simulink model "DCM_Due"  (R2020a)
settings: Solver=FixedStepAuto  StartTime=0.0  StopTime=10  RelTol=1e-3  EnableMultiTasking=on
undefined symbols (not defined in the file): Iumax, J, Ki_I, Kp_I, Kp_W, Kphi, Lu, Ru, T, Ubat
libraries: arduinolib x12, simulink x8, powerlib_meascontrol x1
settings Model: SimulationMode=external  SILPILModeSetting=veronly  ExtModeTrigDuration=2  Creator=Nguyen Tung  LastModifiedBy=Nguyen Tung
settings OptimizationCC: StrengthReduction=on  PassReuseOutputArgsAs=Individual arguments  ZeroExternalMemoryAtStartup=off  ZeroInternalMemoryAtStartup=off  MaxStackSize=64  OptimizeBlockOrder=speed  OptimizationPriority=Speed  OptimizationCustomize=off  MultiThreadedLoops=on  EfficientTunableParamExpr=on
settings DebuggingCC: ParameterTunabilityLossMsg=error
settings HardwareCC: ProdBitPerPointer=32  ProdBitPerSizeT=32  ProdBitPerPtrDiffT=32  ProdLargestAtomicInteger=Long  ProdLargestAtomicFloat=Double  ProdWordSize=32  ProdHWDeviceType=ARM Compatible->ARM Cortex
settings SFSimCC: MATLABDynamicMemAlloc=off
settings RTWCC: SystemTargetFile=ert.tlc  HardwareBoard=Arduino Due  TLCOptions=-aInlineSetEventsForThisBaseRateFcn=TLC_FALSE -aSuppressMultiTaskScheduler=TLC_FALSE -aRateBasedStepFcn=1  TemplateMakefile=ert_default_tmf  GenerateReport=on  Toolchain=Arduino ARM  BuildConfiguration=Faster Runs
settings CodeAppCC: ForceParamTrailComments=on  IgnoreCustomStorageClasses=off  OperatorAnnotations=on  SimulinkDataObjDesc=on  SFDataObjDesc=on  InsertBlockDesc=on
settings ERTTargetCC: SupportContinuousTime=on  SupportVariableSizeSignals=on  ExtMode=on  ExtModeTransport=3  ExtModeStaticAlloc=on  ExtModeStaticAllocSize=24576  ExtModeMexFile=ext_xcp  ExtModeMexArgs=0 5 115200  ExtModeIntrfLevel=Level2 - Open

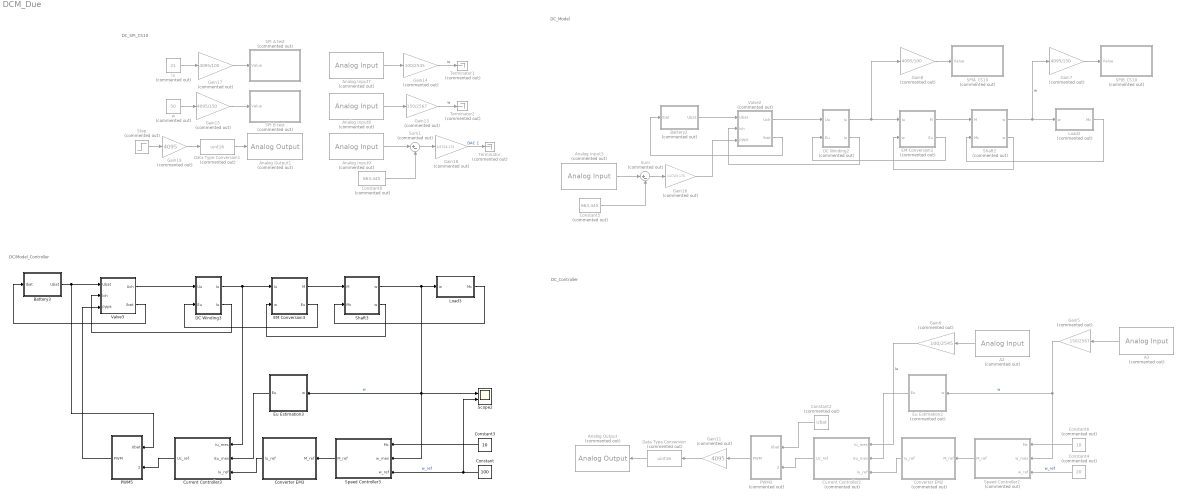
== system DCM_Due ==
  note: DC_Controller
  note: DC/Model_Controller
  note: DC_SPI_CS10
  note: DC_Model
  A2 : arduinolib/Analog Input  Commented=on  pinNumber=2  ReadResultsOnly=off  ConversionTriggerSource=Software  ExternalTriggerType=uint32( 0 )  OutputDataType=uint16  EnableConversionCompleteNotify=off  EnableOuputStatus=off  SampleTime=T  blockPlatform=arduino
  A3 : arduinolib/Analog Input  Commented=on  pinNumber=3  ReadResultsOnly=off  ConversionTriggerSource=Software  ExternalTriggerType=uint32( 0 )  OutputDataType=uint16  EnableConversionCompleteNotify=off  EnableOuputStatus=off  SampleTime=T  blockPlatform=arduino
  Analog Input3 : arduinolib/Analog Input  Commented=on  pinNumber=1  ReadResultsOnly=off  ConversionTriggerSource=Software  ExternalTriggerType=uint32( 0 )  OutputDataType=uint16  EnableConversionCompleteNotify=off  EnableOuputStatus=off  SampleTime=T  blockPlatform=arduino
  Analog Input7 : arduinolib/Analog Input  Commented=on  pinNumber=2  ReadResultsOnly=off  ConversionTriggerSource=Software  ExternalTriggerType=uint32( 0 )  OutputDataType=uint16  EnableConversionCompleteNotify=off  EnableOuputStatus=off  SampleTime=T  blockPlatform=arduino
  Analog Input8 : arduinolib/Analog Input  Commented=on  pinNumber=3  ReadResultsOnly=off  ConversionTriggerSource=Software  ExternalTriggerType=uint32( 0 )  OutputDataType=uint16  EnableConversionCompleteNotify=off  EnableOuputStatus=off  SampleTime=T  blockPlatform=arduino
  Analog Input9 : arduinolib/Analog Input  Commented=on  pinNumber=1  ReadResultsOnly=off  ConversionTriggerSource=Software  ExternalTriggerType=uint32( 0 )  OutputDataType=uint16  EnableConversionCompleteNotify=off  EnableOuputStatus=off  SampleTime=T  blockPlatform=arduino
  Analog Output : arduinolib/Analog Output  Commented=on  DACpin=DAC1  blockPlatform=arduino
      settings: SourceProductBaseCode=ARDUINO
  Analog Output1 : arduinolib/Analog Output  Commented=on  DACpin=DAC1  blockPlatform=arduino
      settings: SourceProductBaseCode=ARDUINO
  Battery2 : Subsystem  Commented=on  AncestorBlock=simulink/REM/SE
      mask Display:
      | plot(0,0,100,100, 1.2*[50,57.68,60.77,63.08,64.97,66.58,68,69.26,70.4, 	71.42,72.36,78.28,80,78.28,72.36,71.42,70.4, 	69.26,68,66.58,64.97,63.08,60.77,57.68,50,42.32, 	39.23,36.92,35.03,33.42,32,30.74,29.6,28.58, 	27.64,21.72,20,21.72,27.64,28.58,29.6,30.74,32, 	33.42,35.03,36.92,39.23,42.32,50]-10, 1.2*[20,21,22,23,24,25,26,27,28,29,30,40,50,60,70,71,72, 	73,74,75,76,77,78,79,80,79,78,77,76,75,74,73,72, 	71,70,60,50,40,30,29,28,27,26,25,24,23,22,21,20]-10)
      | disp('ES')
  Battery3 : Subsystem  AncestorBlock=simulink/REM/SE
      mask Display:
      | plot(0,0,100,100, 1.2*[50,57.68,60.77,63.08,64.97,66.58,68,69.26,70.4, 	71.42,72.36,78.28,80,78.28,72.36,71.42,70.4, 	69.26,68,66.58,64.97,63.08,60.77,57.68,50,42.32, 	39.23,36.92,35.03,33.42,32,30.74,29.6,28.58, 	27.64,21.72,20,21.72,27.64,28.58,29.6,30.74,32, 	33.42,35.03,36.92,39.23,42.32,50]-10, 1.2*[20,21,22,23,24,25,26,27,28,29,30,40,50,60,70,71,72, 	73,74,75,76,77,78,79,80,79,78,77,76,75,74,73,72, 	71,70,60,50,40,30,29,28,27,26,25,24,23,22,21,20]-10)
      | disp('ES')
  Constant : Constant  Value=100  SampleTime=T
  Constant2 : Constant  Commented=on  Value=Ubat
  Constant3 : Constant  Value=10  SampleTime=T
  Constant4 : Constant  Commented=on  Value=20
  Constant5 : Constant  Commented=on  Value=663.445
  Constant6 : Constant  Commented=on  Value=10
  Constant8 : Constant  Commented=on  Value=663.445
  Converter EM2 : Subsystem  Commented=on  AncestorBlock=simulink/SMC/Inversion EC avec mesure
      mask Display: plot(0,0,100,100,[10,30,90,70,10],[90,10,10,90,90])
  Converter EM3 : Subsystem  AncestorBlock=simulink/SMC/Inversion EC avec mesure
      mask Display: plot(0,0,100,100,[10,30,90,70,10],[90,10,10,90,90])
  Current Controller2 : Subsystem  Commented=on  AncestorBlock=simulink/SMC/Asservissement Correcteur IP
      mask Display: plot(0,0,100,100, [10,30,90,70,10,90],[90,10,10,90,90,10])
  Current Controller3 : Subsystem  AncestorBlock=simulink/SMC/Asservissement Correcteur IP
      mask Display: plot(0,0,100,100, [10,30,90,70,10,90],[90,10,10,90,90,10])
  DC Winding2 : Subsystem  Commented=on  AncestorBlock=simulink/REM/EA  mask(CM){}
      mask Display: plot(0,0,100,100,[10,10,90,90,10],[90,10,10,90,90], [10,90],[10,90])
  DC Winding3 : Subsystem  AncestorBlock=simulink/REM/EA  mask(CM){}
      mask Display: plot(0,0,100,100,[10,10,90,90,10],[90,10,10,90,90], [10,90],[10,90])
  Data Type Conversion : DataTypeConversion  Commented=on  OutDataTypeStr=uint16  RndMeth=Nearest
  Data Type Conversion1 : DataTypeConversion  Commented=on  OutDataTypeStr=uint16
  EM Conversion2 : Subsystem  Commented=on  AncestorBlock=simulink/REM/EC EM
      mask Display: plot(0,0,100,100, 1.4*[50,57.68,60.77,63.08,64.97,66.58,68,69.26,70.4, 	71.42,72.36,78.28,80,78.28,72.36,71.42,70.4, 	69.26,68,66.58,64.97,63.08,60.77,57.68,50,42.32, 	39.23,36.92,35.03,33.42,32,30.74,29.6,28.58, 	27.64,21.72,20,21.72,27.64,28.58,29.6,30.74,32, 	33.42,35.03,36.92,39.23,42.32,50]-20, 1.4*[20,21,22,23,24,25,26,27,28,29,30,40,50,60,70,71,72, 	73,74,75,76,77,78,79,80,79,78,77,76,75,74,73,72, 	71,70,60,50,40,30,29,28,27,26,25,24,23,22,21,20]-20)
  EM Conversion3 : Subsystem  AncestorBlock=simulink/REM/EC EM
      mask Display: plot(0,0,100,100, 1.4*[50,57.68,60.77,63.08,64.97,66.58,68,69.26,70.4, 	71.42,72.36,78.28,80,78.28,72.36,71.42,70.4, 	69.26,68,66.58,64.97,63.08,60.77,57.68,50,42.32, 	39.23,36.92,35.03,33.42,32,30.74,29.6,28.58, 	27.64,21.72,20,21.72,27.64,28.58,29.6,30.74,32, 	33.42,35.03,36.92,39.23,42.32,50]-20, 1.4*[20,21,22,23,24,25,26,27,28,29,30,40,50,60,70,71,72, 	73,74,75,76,77,78,79,80,79,78,77,76,75,74,73,72, 	71,70,60,50,40,30,29,28,27,26,25,24,23,22,21,20]-20)
  Eu Estimation2 : Subsystem  Commented=on  AncestorBlock=simulink/REM/EC EM
      mask Display: plot(0,0,100,100, 1.4*[50,57.68,60.77,63.08,64.97,66.58,68,69.26,70.4, 	71.42,72.36,78.28,80,78.28,72.36,71.42,70.4, 	69.26,68,66.58,64.97,63.08,60.77,57.68,50,42.32, 	39.23,36.92,35.03,33.42,32,30.74,29.6,28.58, 	27.64,21.72,20,21.72,27.64,28.58,29.6,30.74,32, 	33.42,35.03,36.92,39.23,42.32,50]-20, 1.4*[20,21,22,23,24,25,26,27,28,29,30,40,50,60,70,71,72, 	73,74,75,76,77,78,79,80,79,78,77,76,75,74,73,72, 	71,70,60,50,40,30,29,28,27,26,25,24,23,22,21,20]-20)
  Eu Estimation3 : Subsystem  AncestorBlock=simulink/REM/EC EM
      mask Display: plot(0,0,100,100, 1.4*[50,57.68,60.77,63.08,64.97,66.58,68,69.26,70.4, 	71.42,72.36,78.28,80,78.28,72.36,71.42,70.4, 	69.26,68,66.58,64.97,63.08,60.77,57.68,50,42.32, 	39.23,36.92,35.03,33.42,32,30.74,29.6,28.58, 	27.64,21.72,20,21.72,27.64,28.58,29.6,30.74,32, 	33.42,35.03,36.92,39.23,42.32,50]-20, 1.4*[20,21,22,23,24,25,26,27,28,29,30,40,50,60,70,71,72, 	73,74,75,76,77,78,79,80,79,78,77,76,75,74,73,72, 	71,70,60,50,40,30,29,28,27,26,25,24,23,22,21,20]-20)
  Gain11 : Gain  Commented=on  Gain=4095
  Gain13 : Gain  Commented=on  Gain=150/2567
  Gain14 : Gain  Commented=on  Gain=100/2545
  Gain15 : Gain  Commented=on  Gain=4095/150
  Gain16 : Gain  Commented=on  Gain=1/2723.175
  Gain17 : Gain  Commented=on  Gain=4095/100
  Gain18 : Gain  Commented=on  Gain=1/2723.175
  Gain19 : Gain  Commented=on  Gain=4095
  Gain5 : Gain  Commented=on  Gain=150/2567
  Gain6 : Gain  Commented=on  Gain=100/2545
  Gain7 : Gain  Commented=on  Gain=4095/150
  Gain8 : Gain  Commented=on  Gain=4095/100
  Iu : Constant  Commented=on  Value=21  SampleTime=T
  Load2 : Subsystem  Commented=on  AncestorBlock=simulink/REM/SE
      mask Display:
      | plot(0,0,100,100, 1.2*[50,57.68,60.77,63.08,64.97,66.58,68,69.26,70.4, 	71.42,72.36,78.28,80,78.28,72.36,71.42,70.4, 	69.26,68,66.58,64.97,63.08,60.77,57.68,50,42.32, 	39.23,36.92,35.03,33.42,32,30.74,29.6,28.58, 	27.64,21.72,20,21.72,27.64,28.58,29.6,30.74,32, 	33.42,35.03,36.92,39.23,42.32,50]-10, 1.2*[20,21,22,23,24,25,26,27,28,29,30,40,50,60,70,71,72, 	73,74,75,76,77,78,79,80,79,78,77,76,75,74,73,72, 	71,70,60,50,40,30,29,28,27,26,25,24,23,22,21,20]-10)
      | disp('MS')
  Load3 : Subsystem  AncestorBlock=simulink/REM/SE
      mask Display:
      | plot(0,0,100,100, 1.2*[50,57.68,60.77,63.08,64.97,66.58,68,69.26,70.4, 	71.42,72.36,78.28,80,78.28,72.36,71.42,70.4, 	69.26,68,66.58,64.97,63.08,60.77,57.68,50,42.32, 	39.23,36.92,35.03,33.42,32,30.74,29.6,28.58, 	27.64,21.72,20,21.72,27.64,28.58,29.6,30.74,32, 	33.42,35.03,36.92,39.23,42.32,50]-10, 1.2*[20,21,22,23,24,25,26,27,28,29,30,40,50,60,70,71,72, 	73,74,75,76,77,78,79,80,79,78,77,76,75,74,73,72, 	71,70,60,50,40,30,29,28,27,26,25,24,23,22,21,20]-10)
      | disp('MS')
  PWM3 : Subsystem  Commented=on  AncestorBlock=simulink/SMC/Inversion EC avec mesure
      mask Display: plot(0,0,100,100,[10,30,90,70,10],[90,10,10,90,90])
  PWM5 : Subsystem  AncestorBlock=simulink/SMC/Inversion EC avec mesure
      mask Display: plot(0,0,100,100,[10,30,90,70,10],[90,10,10,90,90])
  SPI A test : Subsystem  Commented=on
  SPI B test : Subsystem  Commented=on
  SPIA_CS10 : Subsystem  Commented=on
  SPIB_CS10 : Subsystem  Commented=on
  Scope2 : Scope  NumInputPorts=2
  Shaft2 : Subsystem  Commented=on  AncestorBlock=simulink/REM/EA  mask(CM){}
      mask Display: plot(0,0,100,100,[10,10,90,90,10],[90,10,10,90,90], [10,90],[10,90])
  Shaft3 : Subsystem  AncestorBlock=simulink/REM/EA  mask(CM){}
      mask Display: plot(0,0,100,100,[10,10,90,90,10],[90,10,10,90,90], [10,90],[10,90])
  Speed Controller2 : Subsystem  Commented=on  AncestorBlock=simulink/SMC/Asservissement Correcteur IP
      mask Display: plot(0,0,100,100, [10,30,90,70,10,90],[90,10,10,90,90,10])
  Speed Controller3 : Subsystem  AncestorBlock=simulink/SMC/Asservissement Correcteur IP
      mask Display: plot(0,0,100,100, [10,30,90,70,10,90],[90,10,10,90,90,10])
  Step : Step  Commented=on  Time=5  SampleTime=0
  Sum : Sum  Commented=on  Inputs=|+-
  Sum1 : Sum  Commented=on  Inputs=|+-
  Terminator : Terminator  Commented=on
  Terminator1 : Terminator  Commented=on
  Terminator2 : Terminator  Commented=on
  Valve2 : Subsystem  Commented=on  AncestorBlock=simulink/REM/EC Elec  mask(Hacheur){}
      mask Display: plot(0,0,100,100,[10,10,90,90,10],[90,10,10,90,90])
  Valve3 : Subsystem  AncestorBlock=simulink/REM/EC Elec  mask(Hacheur){}
      mask Display: plot(0,0,100,100,[10,10,90,90,10],[90,10,10,90,90])
  w : Constant  Commented=on  Value=50  SampleTime=T
  wires:
  Valve2/1(Uch) -> DC Winding2/1(Uu)
  Speed Controller2/1(M_ref) -> Converter EM2/1(M_ref)
  Valve3/2(Ibat) -> Battery3/1(Ibat)
  A2/1 -> Gain6/1
  Iu/1 -> Gain17/1
  Gain5/1 -> Eu Estimation2/1(w), Speed Controller2/2(w_mes)  "w"
  PWM3/1(PWM) -> Gain11/1
  EM Conversion3/1(M) -> Shaft3/1(M)
  DC Winding2/2("Iu ") -> Valve2/2(Ich)
  Converter EM3/1(Iu_ref) -> Current Controller3/3(Iu_ref)
  Converter EM2/1(Iu_ref) -> Current Controller2/3(Iu_ref)
  Battery3/1(Ubat) -> Valve3/1(Ubat), PWM5/1(Ubat)
  Eu Estimation2/1(Eu) -> Current Controller2/2(Eu_mes)
  Gain16/1 -> Valve2/3(PWM)
  Shaft2/2("w ") -> EM Conversion2/2(w)
  EM Conversion2/2(Eu) -> DC Winding2/2(Eu)
  Analog Input3/1 -> Sum/1
  Gain18/1 -> Terminator/1  "DAC 1"
  Shaft3/1(w) -> Speed Controller3/2(w_mes), Scope2/1, Eu Estimation3/1(w), Load3/1(w)  "w"
  Constant3/1 -> Speed Controller3/1(Mc)
  Gain11/1 -> Data Type Conversion/1
  Speed Controller3/1(M_ref) -> Converter EM3/1(M_ref)
  Current Controller3/1(Uc_ref) -> PWM5/2(Uch_ref)
  DC Winding3/1(Iu) -> EM Conversion3/1(Iu), Current Controller3/1(Iu_mes)
  Data Type Conversion/1 -> Analog Output/1
  Shaft2/1(w) -> Gain7/1, Load2/1(w)  "w"
  PWM5/1(PWM) -> Valve3/3(PWM)
  Constant/1 -> Speed Controller3/3(w_ref), Scope2/2  "w_ref"
  Constant6/1 -> Speed Controller2/1(Mc)
  Step/1 -> Gain19/1
  Data Type Conversion1/1 -> Analog Output1/1
  EM Conversion3/2(Eu) -> DC Winding3/2(Eu)
  Constant8/1 -> Sum1/2
  Gain19/1 -> Data Type Conversion1/1
  A3/1 -> Gain5/1
  Valve2/2(Ibat) -> Battery2/1(Ibat)
  Valve3/1(Uch) -> DC Winding3/1(Uu)
  Constant5/1 -> Sum/2
  DC Winding2/1(Iu) -> Gain8/1, EM Conversion2/1(Iu)
  Constant4/1 -> Speed Controller2/3(w_ref)  "w_ref"
  EM Conversion2/1(M) -> Shaft2/1(M)
  Gain8/1 -> SPIA_CS10/1(Value)
  Load3/1(Mc) -> Shaft3/2(Mc)
  DC Winding3/2("Iu ") -> Valve3/2(Ich)
  Shaft3/2("w ") -> EM Conversion3/2(w)
  Load2/1(Mc) -> Shaft2/2(Mc)
  Gain14/1 -> Terminator1/1  "iu"
  Sum1/1 -> Gain18/1
  Analog Input7/1 -> Gain14/1
  Sum/1 -> Gain16/1
  Gain7/1 -> SPIB_CS10/1(Value)
  Constant2/1 -> PWM3/1(Ubat)
  Analog Input9/1 -> Sum1/1
  Gain17/1 -> SPI A test/1(Value)
  Current Controller2/1(Uc_ref) -> PWM3/2(Uch_ref)
  Battery2/1(Ubat) -> Valve2/1(Ubat)
  Gain6/1 -> Current Controller2/1(Iu_mes)  "Iu"
  Eu Estimation3/1(Eu) -> Current Controller3/2(Eu_mes)
  Gain15/1 -> SPI B test/1(Value)
  Gain13/1 -> Terminator2/1  "w"
  w/1 -> Gain15/1
  Analog Input8/1 -> Gain13/1

== system DCM_Due/Battery2 ==
  Ibat : Inport
  Constant : Constant  Value=Ubat
  Terminator : Terminator
  Ubat : Outport  InitialOutput=0  VectorParamsAs1DForOutWhenUnconnected=off
  wires:
  Constant/1 -> Ubat/1
  Ibat/1 -> Terminator/1

== system DCM_Due/Battery3 ==
  Ibat : Inport
  Constant : Constant  Value=Ubat
  Terminator : Terminator
  Ubat : Outport  InitialOutput=0  VectorParamsAs1DForOutWhenUnconnected=off
  wires:
  Constant/1 -> Ubat/1
  Ibat/1 -> Terminator/1

== system DCM_Due/Converter EM2 ==
  M_ref : Inport
  Gain : Gain  Gain=1/Kphi
  Saturation : Saturate  UpperLimit=Iumax  LowerLimit=0
  Iu_ref : Outport  InitialOutput=0  VectorParamsAs1DForOutWhenUnconnected=off
  wires:
  M_ref/1 -> Gain/1
  Gain/1 -> Saturation/1
  Saturation/1 -> Iu_ref/1

== system DCM_Due/Converter EM3 ==
  M_ref : Inport
  Gain : Gain  Gain=1/Kphi
  Saturation : Saturate  UpperLimit=Iumax  LowerLimit=0
  Iu_ref : Outport  InitialOutput=0  VectorParamsAs1DForOutWhenUnconnected=off
  wires:
  M_ref/1 -> Gain/1
  Gain/1 -> Saturation/1
  Saturation/1 -> Iu_ref/1

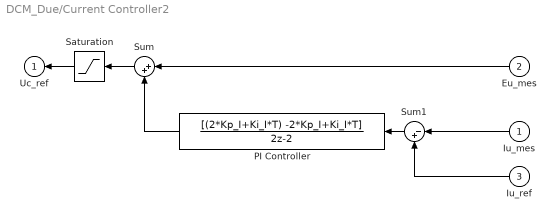
== system DCM_Due/Current Controller2 ==
  Iu_mes : Inport
  Eu_mes : Inport  Port=2
  Iu_ref : Inport  Port=3
  PI Controller : DiscreteTransferFcn  Numerator=[(2*Kp_I+Ki_I*T) -2*Kp_I+Ki_I*T]  Denominator=[2 -2]
  Saturation : Saturate  UpperLimit=Ubat  LowerLimit=0
  Sum : Sum  Inputs=|++
  Sum1 : Sum  Inputs=|-+
  Uc_ref : Outport  InitialOutput=0  VectorParamsAs1DForOutWhenUnconnected=off
  wires:
  Eu_mes/1 -> Sum/1
  Sum/1 -> Saturation/1
  Iu_mes/1 -> Sum1/1
  Sum1/1 -> PI Controller/1
  PI Controller/1 -> Sum/2
  Iu_ref/1 -> Sum1/2
  Saturation/1 -> Uc_ref/1

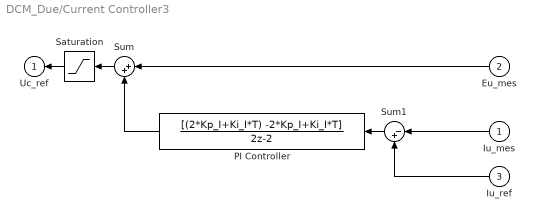
== system DCM_Due/Current Controller3 ==
  Iu_mes : Inport
  Eu_mes : Inport  Port=2
  Iu_ref : Inport  Port=3
  PI Controller : DiscreteTransferFcn  Numerator=[(2*Kp_I+Ki_I*T) -2*Kp_I+Ki_I*T]  Denominator=[2 -2]
  Saturation : Saturate  UpperLimit=Ubat  LowerLimit=0
  Sum : Sum  Inputs=|++
  Sum1 : Sum  Inputs=|-+
  Uc_ref : Outport  InitialOutput=0  VectorParamsAs1DForOutWhenUnconnected=off
  wires:
  Eu_mes/1 -> Sum/1
  Sum/1 -> Saturation/1
  Iu_mes/1 -> Sum1/1
  Sum1/1 -> PI Controller/1
  PI Controller/1 -> Sum/2
  Iu_ref/1 -> Sum1/2
  Saturation/1 -> Uc_ref/1

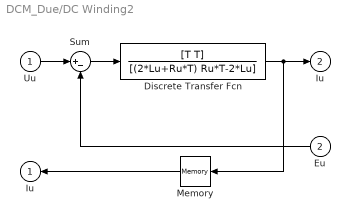
== system DCM_Due/DC Winding2 ==
  Uu : Inport
  Eu : Inport  Port=2
  Discrete Transfer Fcn : DiscreteTransferFcn  Numerator=[T T]  Denominator=[(2*Lu+Ru*T) Ru*T-2*Lu]
  Memory : Memory
  Sum : Sum  Inputs=|+-
  Iu : Outport  InitialOutput=0  VectorParamsAs1DForOutWhenUnconnected=off
  "Iu " : Outport  Port=2  InitialOutput=0  VectorParamsAs1DForOutWhenUnconnected=off
  wires:
  Uu/1 -> Sum/1
  Sum/1 -> Discrete Transfer Fcn/1
  Discrete Transfer Fcn/1 -> Memory/1, "Iu "/1
  Eu/1 -> Sum/2
  Memory/1 -> Iu/1

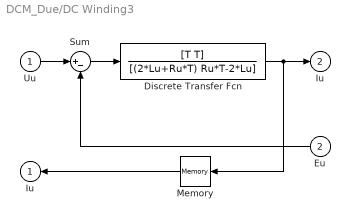
== system DCM_Due/DC Winding3 ==
  Uu : Inport
  Eu : Inport  Port=2
  Discrete Transfer Fcn : DiscreteTransferFcn  Numerator=[T T]  Denominator=[(2*Lu+Ru*T) Ru*T-2*Lu]
  Memory : Memory
  Sum : Sum  Inputs=|+-
  Iu : Outport  InitialOutput=0  VectorParamsAs1DForOutWhenUnconnected=off
  "Iu " : Outport  Port=2  InitialOutput=0  VectorParamsAs1DForOutWhenUnconnected=off
  wires:
  Uu/1 -> Sum/1
  Sum/1 -> Discrete Transfer Fcn/1
  Discrete Transfer Fcn/1 -> Memory/1, "Iu "/1
  Eu/1 -> Sum/2
  Memory/1 -> Iu/1

== system DCM_Due/EM Conversion2 ==
  Iu : Inport
  w : Inport  Port=2
  Gain : Gain  Gain=Kphi
  Gain1 : Gain  Gain=Kphi
  M : Outport  InitialOutput=0  VectorParamsAs1DForOutWhenUnconnected=off
  Eu : Outport  Port=2  InitialOutput=0  VectorParamsAs1DForOutWhenUnconnected=off
  wires:
  Iu/1 -> Gain/1
  Gain/1 -> M/1
  w/1 -> Gain1/1
  Gain1/1 -> Eu/1

== system DCM_Due/EM Conversion3 ==
  Iu : Inport
  w : Inport  Port=2
  Gain : Gain  Gain=Kphi
  Gain1 : Gain  Gain=Kphi
  M : Outport  InitialOutput=0  VectorParamsAs1DForOutWhenUnconnected=off
  Eu : Outport  Port=2  InitialOutput=0  VectorParamsAs1DForOutWhenUnconnected=off
  wires:
  Iu/1 -> Gain/1
  Gain/1 -> M/1
  w/1 -> Gain1/1
  Gain1/1 -> Eu/1

== system DCM_Due/Eu Estimation2 ==
  w : Inport
  Gain1 : Gain  Gain=Kphi
  Eu : Outport  InitialOutput=0  VectorParamsAs1DForOutWhenUnconnected=off
  wires:
  w/1 -> Gain1/1
  Gain1/1 -> Eu/1

== system DCM_Due/Eu Estimation3 ==
  w : Inport
  Gain1 : Gain  Gain=Kphi
  Eu : Outport  InitialOutput=0  VectorParamsAs1DForOutWhenUnconnected=off
  wires:
  w/1 -> Gain1/1
  Gain1/1 -> Eu/1

== system DCM_Due/Load2 ==
  w : Inport
  Step : Step  Time=10  After=10  SampleTime=T
  Terminator : Terminator
  Mc : Outport  InitialOutput=0  VectorParamsAs1DForOutWhenUnconnected=off
  wires:
  w/1 -> Terminator/1
  Step/1 -> Mc/1

== system DCM_Due/Load3 ==
  w : Inport
  Load : Step  Time=5  After=10  SampleTime=T
  Terminator : Terminator
  Mc : Outport  InitialOutput=0  VectorParamsAs1DForOutWhenUnconnected=off
  wires:
  w/1 -> Terminator/1
  Load/1 -> Mc/1

== system DCM_Due/PWM3 ==
  Ubat : Inport
  Uch_ref : Inport  Port=2
  Divide : Product  Inputs=/*
  Gain : Gain  Commented=through  Gain=255
  PWM : Outport
  wires:
  Divide/1 -> Gain/1
  Ubat/1 -> Divide/1
  Uch_ref/1 -> Divide/2
  Gain/1 -> PWM/1

== system DCM_Due/PWM5 ==
  Ubat : Inport
  Uch_ref : Inport  Port=2
  Divide : Product  Inputs=/*
  PWM Generator (DC-DC) : powerlib_meascontrol/Pulse & Signal Generators/PWM Generator (DC-DC)  Commented=through  Fsw=5000  Ts=0
  PWM : Outport
  wires:
  PWM Generator (DC-DC)/1 -> PWM/1
  Ubat/1 -> Divide/1
  Uch_ref/1 -> Divide/2
  Divide/1 -> PWM Generator (DC-DC)/1

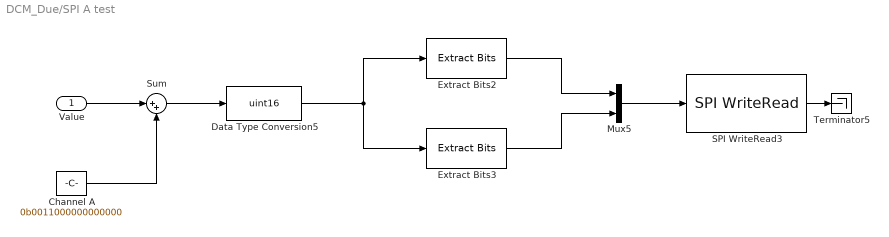
== system DCM_Due/SPI A test ==
  Value : Inport
  Channel A : Constant  Value=0b0011000000000000
  Data Type Conversion5 : DataTypeConversion  OutDataTypeStr=uint16  RndMeth=Nearest
  Extract Bits2 : simulink/Logic and Bit Operations/Extract Bits  bitsToExtract=Range starting with most significant bit  numBits=8  bitIdxRange=[0 7]  outScalingMode=Treat bit field as an integer
  Extract Bits3 : simulink/Logic and Bit Operations/Extract Bits  bitsToExtract=Range ending with least significant bit  numBits=8  bitIdxRange=[0 7]  outScalingMode=Treat bit field as an integer
  Mux5 : Mux  Inputs=2
  SPI WriteRead3 : arduinolib/SPI WriteRead  slaveSelectPin_=10  blockPlatform=arduino
      settings: SourceProductBaseCode=ARDUINO
  Sum : Sum  Inputs=|++
  Terminator5 : Terminator
  wires:
  Extract Bits3/1 -> Mux5/2
  Mux5/1 -> SPI WriteRead3/1
  Channel A/1 -> Sum/2
  Extract Bits2/1 -> Mux5/1
  Data Type Conversion5/1 -> Extract Bits2/1, Extract Bits3/1
  SPI WriteRead3/1 -> Terminator5/1
  Sum/1 -> Data Type Conversion5/1
  Value/1 -> Sum/1

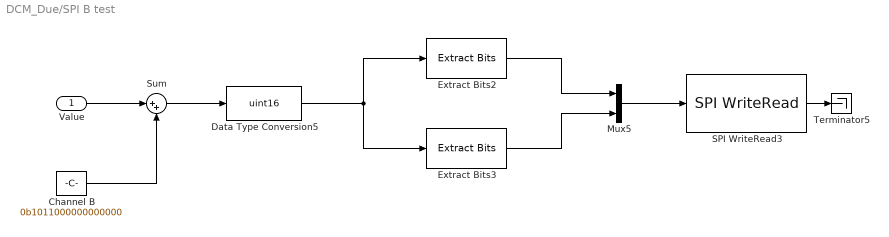
== system DCM_Due/SPI B test ==
  Value : Inport
  Channel B : Constant  Value=0b1011000000000000
  Data Type Conversion5 : DataTypeConversion  OutDataTypeStr=uint16  RndMeth=Nearest
  Extract Bits2 : simulink/Logic and Bit Operations/Extract Bits  bitsToExtract=Range starting with most significant bit  numBits=8  bitIdxRange=[0 7]  outScalingMode=Treat bit field as an integer
  Extract Bits3 : simulink/Logic and Bit Operations/Extract Bits  bitsToExtract=Range ending with least significant bit  numBits=8  bitIdxRange=[0 7]  outScalingMode=Treat bit field as an integer
  Mux5 : Mux  Inputs=2
  SPI WriteRead3 : arduinolib/SPI WriteRead  slaveSelectPin_=10  blockPlatform=arduino
      settings: SourceProductBaseCode=ARDUINO
  Sum : Sum  Inputs=|++
  Terminator5 : Terminator
  wires:
  Extract Bits3/1 -> Mux5/2
  Mux5/1 -> SPI WriteRead3/1
  Channel B/1 -> Sum/2
  Extract Bits2/1 -> Mux5/1
  Data Type Conversion5/1 -> Extract Bits2/1, Extract Bits3/1
  SPI WriteRead3/1 -> Terminator5/1
  Sum/1 -> Data Type Conversion5/1
  Value/1 -> Sum/1

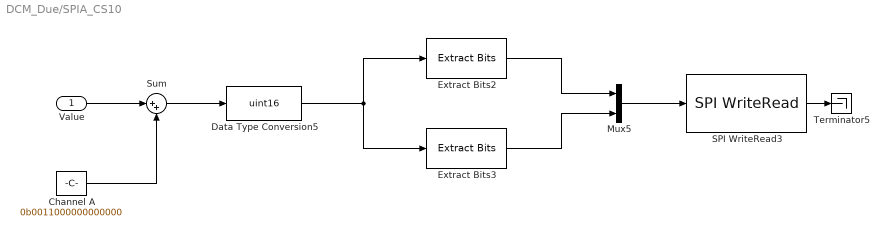
== system DCM_Due/SPIA_CS10 ==
  Value : Inport
  Channel A : Constant  Value=0b0011000000000000
  Data Type Conversion5 : DataTypeConversion  OutDataTypeStr=uint16  RndMeth=Nearest
  Extract Bits2 : simulink/Logic and Bit Operations/Extract Bits  bitsToExtract=Range starting with most significant bit  numBits=8  bitIdxRange=[0 7]  outScalingMode=Treat bit field as an integer
  Extract Bits3 : simulink/Logic and Bit Operations/Extract Bits  bitsToExtract=Range ending with least significant bit  numBits=8  bitIdxRange=[0 7]  outScalingMode=Treat bit field as an integer
  Mux5 : Mux  Inputs=2
  SPI WriteRead3 : arduinolib/SPI WriteRead  slaveSelectPin_=10  blockPlatform=arduino
      settings: SourceProductBaseCode=ARDUINO
  Sum : Sum  Inputs=|++
  Terminator5 : Terminator
  wires:
  Extract Bits3/1 -> Mux5/2
  Mux5/1 -> SPI WriteRead3/1
  Channel A/1 -> Sum/2
  Extract Bits2/1 -> Mux5/1
  Data Type Conversion5/1 -> Extract Bits2/1, Extract Bits3/1
  SPI WriteRead3/1 -> Terminator5/1
  Sum/1 -> Data Type Conversion5/1
  Value/1 -> Sum/1

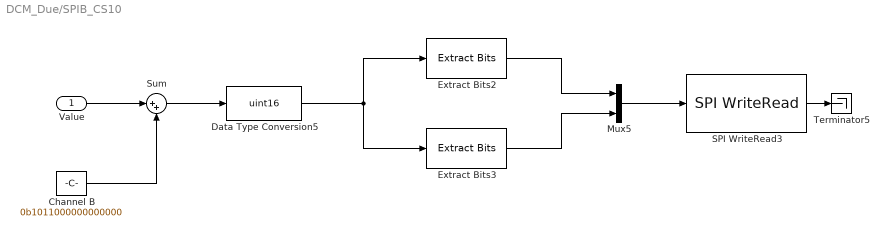
== system DCM_Due/SPIB_CS10 ==
  Value : Inport
  Channel B : Constant  Value=0b1011000000000000
  Data Type Conversion5 : DataTypeConversion  OutDataTypeStr=uint16  RndMeth=Nearest
  Extract Bits2 : simulink/Logic and Bit Operations/Extract Bits  bitsToExtract=Range starting with most significant bit  numBits=8  bitIdxRange=[0 7]  outScalingMode=Treat bit field as an integer
  Extract Bits3 : simulink/Logic and Bit Operations/Extract Bits  bitsToExtract=Range ending with least significant bit  numBits=8  bitIdxRange=[0 7]  outScalingMode=Treat bit field as an integer
  Mux5 : Mux  Inputs=2
  SPI WriteRead3 : arduinolib/SPI WriteRead  slaveSelectPin_=10  blockPlatform=arduino
      settings: SourceProductBaseCode=ARDUINO
  Sum : Sum  Inputs=|++
  Terminator5 : Terminator
  wires:
  Extract Bits3/1 -> Mux5/2
  Mux5/1 -> SPI WriteRead3/1
  Channel B/1 -> Sum/2
  Extract Bits2/1 -> Mux5/1
  Data Type Conversion5/1 -> Extract Bits2/1, Extract Bits3/1
  SPI WriteRead3/1 -> Terminator5/1
  Sum/1 -> Data Type Conversion5/1
  Value/1 -> Sum/1

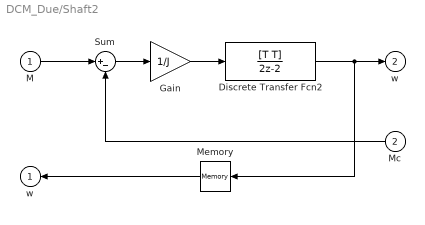
== system DCM_Due/Shaft2 ==
  M : Inport
  Mc : Inport  Port=2
  Discrete Transfer Fcn2 : DiscreteTransferFcn  Numerator=[T T]  Denominator=[2 -2]
  Gain : Gain  Gain=1/J
  Memory : Memory
  Sum : Sum  Inputs=|+-
  w : Outport  InitialOutput=0  VectorParamsAs1DForOutWhenUnconnected=off
  "w " : Outport  Port=2  InitialOutput=0  VectorParamsAs1DForOutWhenUnconnected=off
  wires:
  M/1 -> Sum/1
  Mc/1 -> Sum/2
  Sum/1 -> Gain/1
  Discrete Transfer Fcn2/1 -> Memory/1, "w "/1
  Gain/1 -> Discrete Transfer Fcn2/1
  Memory/1 -> w/1

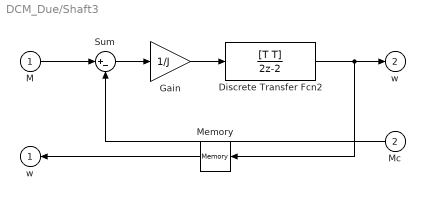
== system DCM_Due/Shaft3 ==
  M : Inport
  Mc : Inport  Port=2
  Discrete Transfer Fcn2 : DiscreteTransferFcn  Numerator=[T T]  Denominator=[2 -2]
  Gain : Gain  Gain=1/J
  Memory : Memory
  Sum : Sum  Inputs=|+-
  w : Outport  InitialOutput=0  VectorParamsAs1DForOutWhenUnconnected=off
  "w " : Outport  Port=2  InitialOutput=0  VectorParamsAs1DForOutWhenUnconnected=off
  wires:
  M/1 -> Sum/1
  Mc/1 -> Sum/2
  Sum/1 -> Gain/1
  Discrete Transfer Fcn2/1 -> Memory/1, "w "/1
  Gain/1 -> Discrete Transfer Fcn2/1
  Memory/1 -> w/1

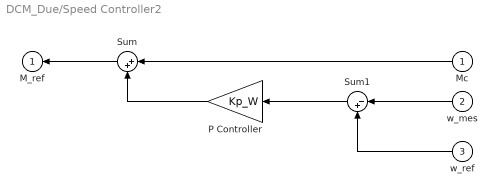
== system DCM_Due/Speed Controller2 ==
  Mc : Inport
  w_mes : Inport  Port=2
  w_ref : Inport  Port=3
  P Controller : Gain  Gain=Kp_W
  Sum : Sum  Inputs=|++
  Sum1 : Sum  Inputs=|-+
  M_ref : Outport  InitialOutput=0  VectorParamsAs1DForOutWhenUnconnected=off
  wires:
  Sum/1 -> M_ref/1
  w_ref/1 -> Sum1/2
  Sum1/1 -> P Controller/1
  P Controller/1 -> Sum/2
  Mc/1 -> Sum/1
  w_mes/1 -> Sum1/1

== system DCM_Due/Speed Controller3 ==
  Mc : Inport
  w_mes : Inport  Port=2
  w_ref : Inport  Port=3
  Gain : Gain  Gain=Kp_W
  Sum : Sum  Inputs=|++
  Sum1 : Sum  Inputs=|-+
  M_ref : Outport  InitialOutput=0  VectorParamsAs1DForOutWhenUnconnected=off
  wires:
  Sum/1 -> M_ref/1
  w_ref/1 -> Sum1/2
  Sum1/1 -> Gain/1
  Gain/1 -> Sum/2
  Mc/1 -> Sum/1
  w_mes/1 -> Sum1/1

== system DCM_Due/Valve2 ==
  Ubat : Inport
  Ich : Inport  Port=2
  PWM : Inport  Port=3
  Product : Product
  Product1 : Product
  Uch : Outport  InitialOutput=0  VectorParamsAs1DForOutWhenUnconnected=off
  Ibat : Outport  Port=2  InitialOutput=0  VectorParamsAs1DForOutWhenUnconnected=off
  wires:
  Product/1 -> Uch/1
  Ubat/1 -> Product/1
  PWM/1 -> Product1/2, Product/2
  Ich/1 -> Product1/1
  Product1/1 -> Ibat/1

== system DCM_Due/Valve3 ==
  Ubat : Inport
  Ich : Inport  Port=2
  PWM : Inport  Port=3
  Product : Product
  Product1 : Product
  Uch : Outport  InitialOutput=0  VectorParamsAs1DForOutWhenUnconnected=off
  Ibat : Outport  Port=2  InitialOutput=0  VectorParamsAs1DForOutWhenUnconnected=off
  wires:
  Product/1 -> Uch/1
  Ubat/1 -> Product/1
  PWM/1 -> Product1/2, Product/2
  Ich/1 -> Product1/1
  Product1/1 -> Ibat/1
